simulink library "vechicleBodyLib"  (R2023b)
settings: Solver=VariableStepAuto  StartTime=0.0  StopTime=10.0  RelTol=1e-3
settings Model: Creator=Madhu B  LastModifiedBy=Madhu B

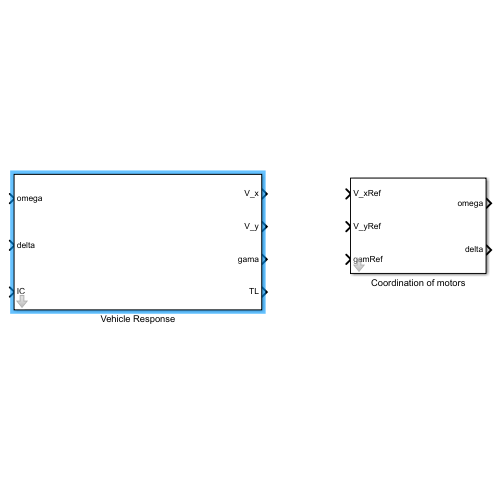
[thumbnail: Simulink's stored preview of the top-level diagram]
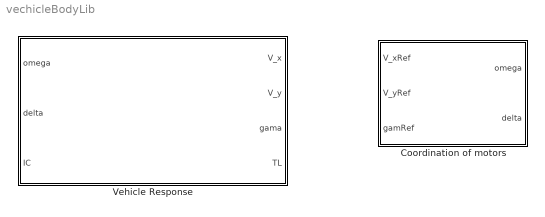
== system vechicleBodyLib ==
  Coordination of motors : Subsystem  mask{r=1, lf=0, lr=0, ld=0}
      mask prompts: r "Radius of wheel"; lf "CM location from front wheel(lf)"; lr "CM location from rear wheel(lr)"; ld "half of track(ld)"
      mask DialogControl DescTextVar Prompt: Eight motor coordinator
      mask DialogControl vc Prompt: Radius of wheel
  Vehicle Response : Subsystem  mask{M=1, Jm=0.5, h=0, ld=0, lf=0, lr=0, Kf=0, Kr=0, r=0}
      mask prompts: M "Mass"; Jm "Moment of inertia"; h "Center of mass height(h)"; ld "half of track(ld)"; lf "CM location from front wheel(lf)"; lr "CM location from rear wheel(lr)"; Kf "Front suspension stiffness"; Kr "Rear suspension stiffness"; r "Radius of wheel"
      mask DialogControl DescGroupVar Prompt: Vechicle body Response
      mask DialogControl DescTextVar Prompt: Enter the vechicle parameters.
      mask DialogControl Control2 Prompt: Create a fucntion uRes

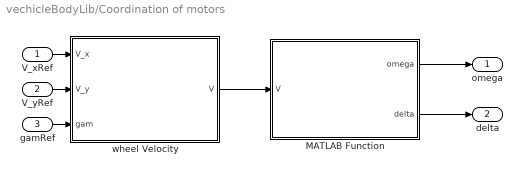
== system vechicleBodyLib/Coordination of motors ==
  V_xRef : Inport
  V_yRef : Inport  Port=2
  gamRef : Inport  Port=3
  MATLAB Function : MATLAB Function  TreatAsAtomicUnit=on
  wheel Velocity : MATLAB Function  TreatAsAtomicUnit=on
  omega : Outport
  delta : Outport  Port=2
  wires:
  V_xRef/1 -> wheel Velocity/1(V_x)
  V_yRef/1 -> wheel Velocity/2(V_y)
  gamRef/1 -> wheel Velocity/3(gam)
  wheel Velocity/1(V) -> MATLAB Function/1(V)
  MATLAB Function/1(omega) -> omega/1
  MATLAB Function/2(delta) -> delta/1

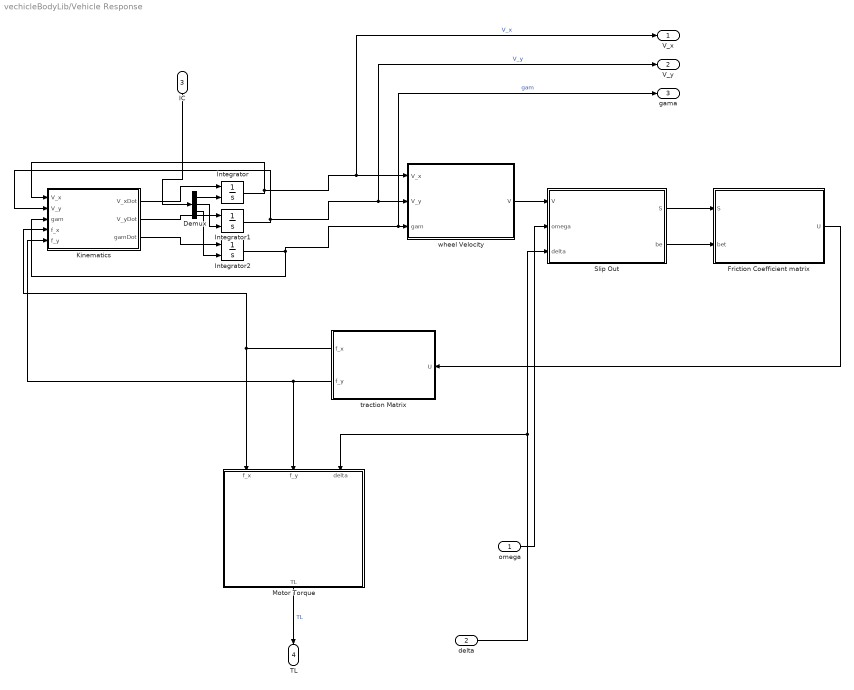
== system vechicleBodyLib/Vehicle Response ==
  omega : Inport
  delta : Inport  Port=2
  IC : Inport  Port=3
  " Friction Coefficient matrix" : MATLAB Function  TreatAsAtomicUnit=on
  Demux : Demux  Outputs=3
  Integrator : Integrator  InitialConditionSource=external
  Integrator1 : Integrator  InitialConditionSource=external
  Integrator2 : Integrator  InitialConditionSource=external
  Kinematics : MATLAB Function  TreatAsAtomicUnit=on
  Motor Torque : MATLAB Function  TreatAsAtomicUnit=on
  Slip Out : MATLAB Function  TreatAsAtomicUnit=on
  traction Matrix : MATLAB Function  TreatAsAtomicUnit=on
  wheel Velocity : MATLAB Function  TreatAsAtomicUnit=on
  V_x : Outport
  V_y : Outport  Port=2
  gama : Outport  Port=3
  TL : Outport  Port=4
  wires:
  delta/1 -> Motor Torque/3(delta), Slip Out/3(delta)
  traction Matrix/2(f_y) -> Kinematics/5(f_y), Motor Torque/2(f_y)
  omega/1 -> Slip Out/2(omega)
  wheel Velocity/1(V) -> Slip Out/1(V)
  Slip Out/1(S) -> " Friction Coefficient matrix"/1(S)
  " Friction Coefficient matrix"/1(U) -> traction Matrix/1(U)
  traction Matrix/1(f_x) -> Kinematics/4(f_x), Motor Torque/1(f_x)
  Slip Out/2(be) -> " Friction Coefficient matrix"/2(bet)
  Motor Torque/1(TL) -> TL/1  "TL"
  Kinematics/1(V_xDot) -> Integrator/1
  Kinematics/2(V_yDot) -> Integrator1/1
  Kinematics/3(gamDot) -> Integrator2/1
  Integrator/1 -> Kinematics/1(V_x), V_x/1, wheel Velocity/1(V_x)  "V_x"
  Integrator1/1 -> Kinematics/2(V_y), V_y/1, wheel Velocity/2(V_y)  "V_y"
  Integrator2/1 -> gama/1, wheel Velocity/3(gam), Kinematics/3(gam)  "gam"
  Demux/1 -> Integrator/2
  Demux/2 -> Integrator1/2
  Demux/3 -> Integrator2/2
  IC/1 -> Demux/1

== matlab function vechicleBodyLib/Coordination of motors/MATLAB Function ==
  data: V input; omega output; delta output; r parameter
function [omega,delta] = motIn(V,r)
omega=[1;1;1;1]; delta=omega;
for i=1:4
   omega(i)=norm(V(:,i))/r;
   delta(i)=atan2(V(2,i),V(1,i));
end
end

== matlab function vechicleBodyLib/Vehicle Response/Kinematics ==
  data: V_xDot output size=1; V_yDot output size=1; V_x input; V_y input; gam input; ld parameter; lr parameter; lf parameter; M parameter; Jm parameter; f_x input size=[4 1]; gamDot output size=1; f_y input size=[4 1]
function [V_xDot,V_yDot,gamDot] = kine( V_x,V_y,gam,ld, lr, lf, M, Jm,f_x,f_y)
S=ld*(f_x(2)+f_x(4)-(f_x(1)+f_x(3)));
S=S+lf*(f_y(1)+f_y(2))-lr*(f_y(3)+f_y(4));
gamDot=S/Jm;
E=sum(f_x)+M*gam*V_y;
V_xDot=E/M;
E=sum(f_y)-M*gam*V_x;
V_yDot=E/M;
end

== matlab function vechicleBodyLib/Coordination of motors/wheel Velocity ==
  data: V_x input size=1; V output size=[2 4]; V_y input size=1; gam input size=1; ld parameter size=1; lf parameter size=1; lr parameter size=1
function V = wheel(V_x,V_y,gam,ld, lf, lr)
S=[V_x-ld*gam V_x+ld*gam V_x-ld*gam V_x+ld*gam;
    V_y+lf*gam V_y+lf*gam V_y-lr*gam V_y-lr*gam];
V=S;
end

== matlab function vechicleBodyLib/Vehicle Response/wheel Velocity ==
  data: V_x input; V output; V_y input; gam input; ld parameter; lf parameter; lr parameter
function V = wheel(V_x,V_y,gam,ld, lf, lr)
S=[V_x-ld*gam V_x+ld*gam V_x-ld*gam V_x+ld*gam;
    V_y+lf*gam V_y+lf*gam V_y-lr*gam V_y-lr*gam];
V=S;
end

== matlab function vechicleBodyLib/Vehicle Response/Slip Out ==
  data: V input; S output; omega input; delta input; be output; r parameter
function [S,be] = Sout(V,omega,delta,r)

D=V;
be=[1 1 1 1];
for i=1:4
D(:,i)=slip(D(:,i),i);
end    
S=D;
function [Sj] = slip(v,i)
be(i)=atan2(v(2),v(1));
alp=delta(i)-be(i);
Sjx=r*omega(i)*cos(alp);
Df=max([Sjx norm(v)]);
if(Df==0)
    Sj=[0;0];
else
Sjx=(r*omega(i)*cos(alp)-norm(v))/Df;
Sjy=r*omega(i)*sin(alp)/Df;
Sj=[Sjx ; Sjy];
end
end
end

== matlab function vechicleBodyLib/Vehicle Response/ Friction Coefficient matrix ==
  data: S input; U output; bet input
function U = fric(S,bet)
X=S;
for i=1:4
X(:,i)=fric(i);
end
U=X;
function Q = fric(i)
A=[cos(bet(i)) -sin(bet(i));sin(bet(i)) cos(bet(i))];
S_i=S(:,i);
modS_i=norm(S_i);
if modS_i==0
    Q=[0 ;0];
else
mew=uRes(modS_i);
W=(mew/modS_i)*S_i;
Q=A*W;
end
end
end

== matlab function vechicleBodyLib/Vehicle Response/traction Matrix ==
  data: U input; f_x output size=[4 1]; f_y output size=[4 1]; ld parameter; lr parameter; lf parameter; h parameter; M parameter; Kf parameter; Kr parameter
function [f_x, f_y] = traction(U,ld, lr, lf, h, M,Kf, Kr)
g=9.81;
L=lr+lf;
K=Kf+Kr;
Fzs=M*g/2*[lr/L ;lr/L ;lf/L ;lf/L];
G=[h/(2*L) (Kf*h)/(2*K*ld);
   h/(2*L) (-Kf*h)/(2*K*ld);
   -h/(2*L) (Kr*h)/(2*K*ld);
   -h/(2*L) (-Kr*h)/(2*K*ld)];
T=(eye(4))+(G*U);
Fz=T\Fzs;
N=U;
for i=1:4
N(:,i)=N(:,i)*Fz(i);
end
    f_x=N(1,:)';
    f_y=N(2,:)';
end

== matlab function vechicleBodyLib/Vehicle Response/Motor Torque ==
  data: f_x input; TL output; f_y input; delta input; r parameter
function TL = motTorque(f_x,f_y,delta,r)
TL=zeros(4,1);
for i=1:4
    TL(i)=(f_x(i)*r*cos(delta(i)))+(f_y(i)*r*sin(delta(i)));
end
end
